simulink model "aerosonde_trim"  (Simulink 7.5)
settings: Solver=ode3  StartTime=0.0  StopTime=60  FixedStep=20e-3  RelTol=1e-6
values from neighbouring files (symbols this model uses):
  aerosonde = aerosonde_data    [aerosonde_initialize.m]    (also in aerosonde_trimlin.m)
  euler_ini = [0;  0.0564; 0]    [aerosonde_trimlin.m]
  fuel_ini = 2    [aerosonde_trimlin.m]
  Omega_ini = 5236*pi/30    (= 548.312637807)    [aerosonde_trimlin.m]
  position_ini = [0; 0; -1000]    [aerosonde_trimlin.m]
  rates_ini = [0; 0; 0]    [aerosonde_trimlin.m]
  velocity_ini = [24.95;   0;   1.4]    [aerosonde_trimlin.m]
libraries: aerolibasang x3, aerolibbdyn x3, aerolibadyn x1, aerolibtransform2 x1, aerolib6dof2 x1, aerolibutil x1, aerolibatmos2 x1
settings Model: Creator=eh3081  LastModifiedBy=eh3081
settings DataIOCC: LimitDataPoints=off  SaveOutput=off  SignalLogging=off  SaveTime=off
settings OptimizationCC: InitFltsAndDblsToZero=on
settings DebuggingCC: SaveWithParameterizedLinksMsg=none  MultiTaskDSMMsg=warning  MultiTaskCondExecSysMsg=none  StrictBusMsg=Warning
settings RTWCC: IncludeERTFirstTime=on
settings GRTTargetCC: TargetFcnLib=ansi_tfl_tmw.mat

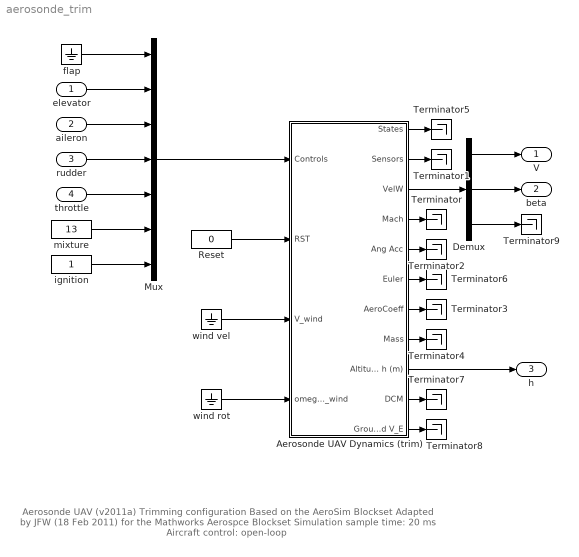
== system aerosonde_trim ==
  note: Aerosonde UAV (v2011a)
      | Trimming configuration
      | Based on the AeroSim Blockset
      | Adapted by JFW (18 Feb 2011) for the Mathworks Aerospce Blockset
      | Simulation sample time: 20 ms
      | Aircraft control: open-loop
  elevator : Inport
  aileron : Inport  Port=2
  rudder : Inport  Port=3
  throttle : Inport  Port=4
  Aerosonde UAV Dynamics (trim) : Subsystem  mask(6-DOF Aerosonde Model){as=aerosonde, Velocities0=velocity_ini, Rates0=rates_ini, Euler0=euler_ini, Position0=position_ini, Fuel0=fuel_ini, Omega0=Omega_ini, GndAlt=0}
      mask prompts: as "Aircraft configuration data:"; Velocities0 "Initial velocity in body axes [u,v,w]: (m/s)"; Rates0 "Initial body rotation rates [p,q,r]: (rad/s)"; Euler0 "Initial Euler orientation [roll, pitch, yaw]: (rad)"; Position0 "Initial position in inertial axes [Xe,Ye,Ze]: (m)"; Fuel0 "Initial fuel mass: (Kg)"; Omega0 "Initial engine speed: (rad/s)"; GndAlt "Ground altitude: (m)"
      mask help:
      | Nonlinear 6-DOF Aerosonde  model with equations of motion in
      | body frame (trim).
      |
      | Version 2011a (18 February 2011)
      |
      | NOTE: the algebraic loop has been removed and the rate set to zero
      |       the wind rate has been set to zero
      mask Help:
      | The block implements the 6-DOF nonlinear Aerosonde model. It is an adaptation of the model provided in the AeroSim blockset. Velocities are computed in body frame.
      | <P><B>Inputs:</B>
      | <LI>Controls = the 4x1 vector of aircraft controls [elevator aileron rudder throttle]. Aerodynamic controls are in radians, throttle is from 0 to 1.</LI>
      | <LI>RST = the integrator reset flag (0 or 1, all integrators on rising edge)
      | <LI>V_wind = the 3x1 vector of background wind speed components in navigation frame [North East Down]</LI>
      | <LI>omega_wind = the 3x1 vector of background wind angular rates in navigation frame [North East Down]</LI>
      | </P>
      | <P><B>Outputs:</B>
      | <LI>States = the 14x1 aircraft state vector [Velocities, Angular rates, Euler angles, Position, Fuel mass, Engine speed].</LI>
      | <LI>Sensors = the 15x1 vector of sensor outputs [GPS Position, GPS Groundspeed, Accelerometers, Gyros, Air data].</LI>
      | <LI>VelW = the 3x1 vector of aircraft velocity in wind axes [Airspeed, sideslip, angle of attack]</LI>
      | <LI>Mach = the Mach number</LI>
      | <LI>Ang Acc = the 3x1 vector of angular accelerations
      | <LI>Euler = the 3x1 vector of Euler angles (roll, pitch, yaw)</LI>
      | <LI>AeroCoeff = the 6x1 vector of aerodynamic coefficients [CD CY CL Cl Cm Cn]</LI>
      | <LI>Mass = the current aircraft mass</LI>
      | <LI>h = the aircraft altitude</LI>
      | </P>
      | <P><B>Parameters:</B>
      | <LI>Aircraft configuration data = structured varaible with aircraft data<BR>
      | obtain by  ``aerosonde=aerosonde_initialize'' for example</LI>
      | <LI>Initial velocities = the 3x1 vector of initial aircraft velocities in body axes [u v w]</LI>
      | <LI>Initial angular rates = the 3x1 vector of initial angular rates [p q r]</LI>
      | <LI>Initial attitude = the 3x1 vector of initial Euler angles [phi theta psi]</LI>
      | <LI>Initial position = the 3x1 vector of initial aircraft location [Lat Lon Alt]</LI>
      | <LI>Initial fuel mass = the initial quantity of fuel on-board the aircraft</LI>
      | <LI>Initial engine speed = the initial engine rotation speed</LI>
      | <LI>Ground altitude = the ground altitude at aircraft location</LI>
      | </P>
      | <P>
      | <I>Version 2010b (26 May 2010)</I>
      | </P>
  Demux : Demux  Outputs=3
  Mux : Mux  Inputs=7
  Reset : Constant  Value=0
  Terminator{,1..9} (10 alike) : Terminator
  flap : Ground
  ignition : Constant
  mixture : Constant  Value=13
  wind rot : Ground
  wind vel : Ground
  V : Outport
  beta : Outport  Port=2
  h : Outport  Port=3
  wires:
  Reset/1 -> Aerosonde UAV Dynamics (trim)/2(RST)
  Demux/3 -> Terminator9/1
  Aerosonde UAV Dynamics (trim)/3(VelW) -> Demux/1
  Aerosonde UAV Dynamics (trim)/4(Mach) -> Terminator/1
  Aerosonde UAV Dynamics (trim)/2(Sensors) -> Terminator1/1
  Aerosonde UAV Dynamics (trim)/5(Ang Acc) -> Terminator2/1
  Aerosonde UAV Dynamics (trim)/7(AeroCoeff) -> Terminator3/1
  Aerosonde UAV Dynamics (trim)/8(Mass) -> Terminator4/1
  Aerosonde UAV Dynamics (trim)/1(States) -> Terminator5/1
  Aerosonde UAV Dynamics (trim)/9("Altitude h (m) ") -> h/1
  wind vel/1 -> Aerosonde UAV Dynamics (trim)/3(V_wind)
  wind rot/1 -> Aerosonde UAV Dynamics (trim)/4(omega_wind)
  Aerosonde UAV Dynamics (trim)/6(Euler) -> Terminator6/1
  Aerosonde UAV Dynamics (trim)/10(DCM) -> Terminator7/1
  Aerosonde UAV Dynamics (trim)/11(Groundspeed V_E) -> Terminator8/1
  Mux/1 -> Aerosonde UAV Dynamics (trim)/1(Controls)
  flap/1 -> Mux/1
  elevator/1 -> Mux/2
  aileron/1 -> Mux/3
  rudder/1 -> Mux/4
  throttle/1 -> Mux/5
  mixture/1 -> Mux/6
  ignition/1 -> Mux/7
  Demux/1 -> V/1
  Demux/2 -> beta/1

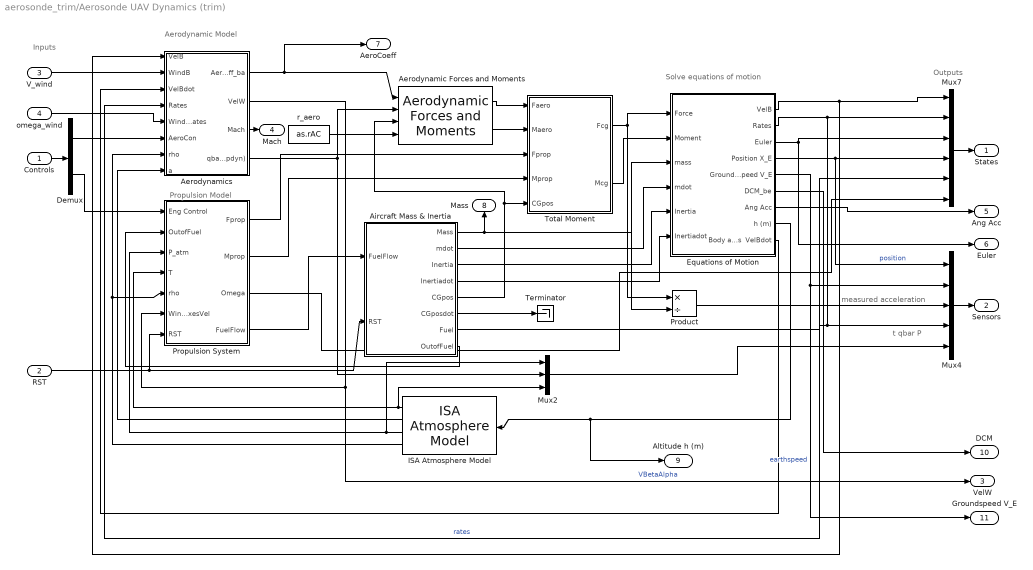
== system aerosonde_trim/Aerosonde UAV Dynamics (trim) ==
  note: Solve equations of motion
  note: Inputs
  note: Outputs
  note: Aerodynamic Model
  note: Propulsion Model
  note: measured acceleration
  note: t qbar P
  Controls : Inport
  RST : Inport  Port=2
  V_wind : Inport  Port=3
  omega_wind : Inport  Port=4
  Aerodynamic Forces and Moments : aerolibadyn/Aerodynamic Forces and Moments   SystemSampleTime=-1  inputAxes=Body  outputForceAxes=Body  outputMomentAxes=Body  S=as.S  b=as.b  cbar=as.c
  Aerodynamics : Subsystem
  Aircraft Mass & Inertia : Subsystem
  Demux : Demux  Outputs=[4,3]
  Equations of Motion : Subsystem
  ISA Atmosphere Model : aerolibatmos2/ISA Atmosphere Model  SystemSampleTime=-1  custom=off  g=9.80665  gamma=1.4  R=287.0531  L=0.0065  h_trop=11000  h_strat=20000  rho0=1.225  P0=101325  T0=288.15
  Mux2 : Mux  Inputs=3
  Mux4 : Mux  Inputs=5
  Mux7 : Mux  Inputs=6
  Product : Product  Inputs=*/  RndMeth=Zero
  Propulsion System : Subsystem  mask(General-aviation propulsion system){OmegaIni=Omega0, RPM=as.RPM, MAP=as.MAP, FuelFlow=as.FuelFlow, Power=as.Power, Jeng=as.Jeng, J=as.J, CT=as.CT, CP=as.CP, Rprop=as.Rprop, Jprop=as.Jprop, TSL=as.TSL}
      mask prompts: OmegaIni "Initial engine speed:"; RPM "Engine RPM vector:"; MAP "Engine MAP vector:"; FuelFlow "Engine fuel flow look-up table:"; Power "Engine power look-up table:"; Jeng "Engine moment of inertia:"; J "Propeller advance ratio vector:"; CT "Propeller coefficient of thrust vector:"; CP "Propeller coefficient of power vector:"; Rprop "Propeller radius:"; Jprop "Propeller moment of inertia:"; TSL "Sea-level temperature:"
      mask help: The block models a general aviation propulsion system including a piston engine and a fixed-pitch propeller.
      mask Help:
      | The block provides a general aviation propulsion system using the AeroSim piston engine and fixed-pitch propeller models.
      | <P><B>Inputs:</B>
      | <LI>Control = the 3x1 engine control vector [Throttle Mixture Ignition]</LI>
      | <LI>OutofFuel = the out-of-fuel flag (0 or 1)</LI>
      | <LI>p = the static pressure at current altitude, in Pa</LI>
      | <LI>T = the air temperature at current altitude, in K</LI>
      | <LI>rho = the air density at current altitude, in kg/m^3</LI>
      | <LI>WindAxesVel = the 3x1 vector of body velocities in wind axes [Airspeed Sideslip Angle-of-attack] in [m/s rad rad]</LI>
      | <LI>RST = the integrator reset flag (rising edge)</LI>
      | </P>
      | <P><B>Output:</B>
      | <LI>Fprop = the 3x1 vector of propulsion system forces applied to the airframe, at the propeller hub location</LI>
      | <LI>Mprop = the 3x1 vector of propulsion system moments applied to the airframe</LI>
      | <LI>Omega = the engine shaft rotation speed, in rad/s</LI>
      | <LI>FuelFlow = the mass fuel flow, in kg/s</LI>
      | <LI>EngCoeff = the 5x1 engine coefficient vector [MAP Airflow Fuelflow BSFC Power] in [kPa kg/s kg/s g/(W*hr) W]</LI>
      | <LI>PropCoeff = the 3x1 propeller coefficient vector [J CT CP]</LI>
      | </P>
      | <P><B>Parameters:</B>
      | <LI>Initial engine speed = the initial value for the engine speed, in rad/s</LI>
      | <LI>RPM vector = the engine speed interpolation vector, in rpm</LI>
      | <LI>MAP vector = the manifold air pressure interpolation vector, in kPa</LI>
      | <LI>Fuel flow = the 2-D look-up table for fuel flow, as function of MAP and RPM, in g/hr</LI>
      | <LI>Power = the 2-D look-up table for power, as function of MAP and RPM, in W</LI>
      | <LI>Engine moment of inertia = the moment of inertia of the rotating engine parts (shaft)</LI>
      | <LI>Advance ratio = the advance ratio vector for interpolation</LI>
      | <LI>Coefficient of thrust = the coefficient of thrust vector for interpolation</LI>
      | <LI>Coefficient of power = the coefficient of power vector for interpolation</LI>
      | <LI>Radius = the propeller radius</LI>
      | <LI>Propeller moment of inertia = the moment of inertia of the propeller</LI>
      | <LI>Sea-level temperature = the ambient temperature for which the above engine look-up tables are given</LI>
      | </P>
  Terminator : Terminator
  Total Moment : Subsystem
  r_aero : Constant  Value=as.rAC
  States : Outport
  Sensors : Outport  Port=2
  VelW : Outport  Port=3
  Mach : Outport  Port=4
  Ang Acc : Outport  Port=5
  Euler : Outport  Port=6
  AeroCoeff : Outport  Port=7
  Mass : Outport  Port=8
  "Altitude h (m) " : Outport  Port=9
  DCM : Outport  Port=10
  Groundspeed V_E : Outport  Port=11
  wires:
  Equations of Motion/3(Euler) -> Euler/1, Mux7/3
  Equations of Motion/7(Ang Acc) -> Ang Acc/1
  RST/1 -> Propulsion System/7(RST), Aircraft Mass & Inertia/2(RST)
  Aircraft Mass & Inertia/8(OutofFuel) -> Propulsion System/2(OutofFuel)
  Aerodynamics/2(VelW) -> Propulsion System/6(WindAxesVel), VelW/1  "VBetaAlpha"
  Propulsion System/3(Omega) -> Mux7/6
  Aircraft Mass & Inertia/7(Fuel) -> Mux7/5
  Mux2/1 -> Mux4/5
  Aerodynamics/4(qbar (pdyn)) -> Mux2/2, Aerodynamic Forces and Moments/2
  Equations of Motion/6(DCM_be) -> DCM/1
  Propulsion System/2(Mprop) -> Total Moment/4(Mprop)
  Propulsion System/1(Fprop) -> Total Moment/3(Fprop)
  Aircraft Mass & Inertia/5(CGpos) -> Total Moment/5(CGpos), Aerodynamic Forces and Moments/3
  Total Moment/2(Mcg) -> Equations of Motion/2(Moment)
  Aircraft Mass & Inertia/1(Mass) -> Mass/1, Equations of Motion/3(mass), Product/2
  Equations of Motion/5(Groundspeed V_E) -> Mux4/2, Groundspeed V_E/1  "earthspeed"
  Controls/1 -> Demux/1
  Mux4/1 -> Sensors/1
  Mux7/1 -> States/1
  Demux/2 -> Propulsion System/1(Eng Control)
  Equations of Motion/1(VelB) -> Mux7/1, Aerodynamics/1(VelB)
  Equations of Motion/2(Rates) -> Aerodynamics/4(Rates), Mux4/4, Mux7/2  "rates"
  Equations of Motion/4(Position X_E) -> Mux7/4, Mux4/1  "position"
  Demux/1 -> Aerodynamics/6(AeroCon)
  Aerodynamics/3(Mach) -> Mach/1
  Aerodynamics/1(AeroCoeff_ba) -> AeroCoeff/1, Aerodynamic Forces and Moments/1
  ISA Atmosphere Model/1 -> Propulsion System/4(T), Mux2/3
  ISA Atmosphere Model/2 -> Aerodynamics/8("a ")
  ISA Atmosphere Model/3 -> Propulsion System/3(P_atm), Mux2/1
  ISA Atmosphere Model/4 -> Aerodynamics/7(rho), Propulsion System/5(rho)
  Equations of Motion/8(h (m)) -> ISA Atmosphere Model/1, "Altitude h (m) "/1
  Aircraft Mass & Inertia/2(mdot) -> Equations of Motion/4(mdot)
  r_aero/1 -> Aerodynamic Forces and Moments/4
  Aerodynamic Forces and Moments/1 -> Total Moment/1(Faero)
  Aerodynamic Forces and Moments/2 -> Total Moment/2(Maero)
  Total Moment/1(Fcg) -> Equations of Motion/1(Force), Product/1
  Aircraft Mass & Inertia/3(Inertia) -> Equations of Motion/5(Inertia)
  Aircraft Mass & Inertia/4(Inertiadot) -> Equations of Motion/6(Inertiadot)
  Aircraft Mass & Inertia/6(CGposdot) -> Terminator/1
  Product/1 -> Mux4/3
  Propulsion System/4(FuelFlow) -> Aircraft Mass & Inertia/1(FuelFlow)
  Equations of Motion/9(Body accns  VelBdot) -> Aerodynamics/3(VelBdot)
  omega_wind/1 -> Aerodynamics/5(WindRates)
  V_wind/1 -> Aerodynamics/2(WindB)

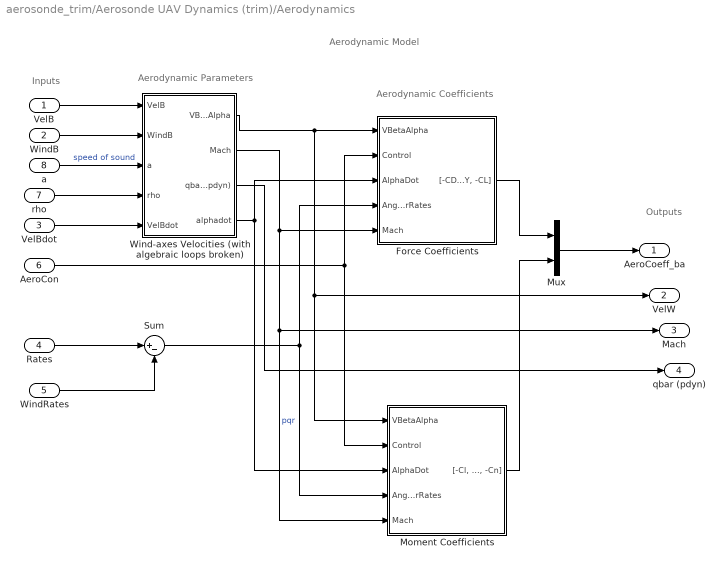
== system aerosonde_trim/Aerosonde UAV Dynamics (trim)/Aerodynamics ==
  note: Inputs
  note: Outputs
  note: Aerodynamic Parameters
  note: Aerodynamic Coefficients
  note: Aerodynamic Model
  VelB : Inport  PortDimensions=[3 1]
  WindB : Inport  Port=2  PortDimensions=[3 1]
  VelBdot : Inport  Port=3
  Rates : Inport  Port=4  PortDimensions=[3 1]
  WindRates : Inport  Port=5  PortDimensions=[3 1]
  AeroCon : Inport  Port=6  PortDimensions=[4 1]
  rho : Inport  Port=7  PortDimensions=1
  "a " : Inport  Port=8  PortDimensions=1
  Force Coefficients : Subsystem
  Moment Coefficients : Subsystem
  Mux : Mux  Inputs=2
  Sum : Sum  Inputs=|+-  SaturateOnIntegerOverflow=on  InputSameDT=on  OutDataTypeStr=Inherit: Same as first input
  Wind-axes Velocities (with algebraic loops broken) : Subsystem
  AeroCoeff_ba : Outport
  VelW : Outport  Port=2
  Mach : Outport  Port=3
  qbar (pdyn) : Outport  Port=4
  wires:
  Sum/1 -> Force Coefficients/4(AngularRates), Moment Coefficients/4(AngularRates)  "pqr"
  WindRates/1 -> Sum/2
  Rates/1 -> Sum/1
  Wind-axes Velocities (with algebraic loops broken)/3(qbar (pdyn)) -> qbar (pdyn)/1
  Wind-axes Velocities (with algebraic loops broken)/2(Mach) -> Mach/1, Force Coefficients/5(Mach), Moment Coefficients/5(Mach)
  AeroCon/1 -> Force Coefficients/2(Control), Moment Coefficients/2(Control)
  Wind-axes Velocities (with algebraic loops broken)/1(VBetaAlpha) -> Force Coefficients/1(VBetaAlpha), VelW/1, Moment Coefficients/1(VBetaAlpha)
  "a "/1 -> Wind-axes Velocities (with algebraic loops broken)/3(a)  "speed of sound"
  VelB/1 -> Wind-axes Velocities (with algebraic loops broken)/1(VelB)
  rho/1 -> Wind-axes Velocities (with algebraic loops broken)/4(rho)
  Force Coefficients/1("[-CD, CY, -CL]") -> Mux/1
  Moment Coefficients/1("[-Cl, Cm, -Cn]") -> Mux/2
  Mux/1 -> AeroCoeff_ba/1
  WindB/1 -> Wind-axes Velocities (with algebraic loops broken)/2(WindB)
  Wind-axes Velocities (with algebraic loops broken)/4(alphadot) -> Moment Coefficients/3(AlphaDot), Force Coefficients/3(AlphaDot)
  VelBdot/1 -> Wind-axes Velocities (with algebraic loops broken)/5(VelBdot)

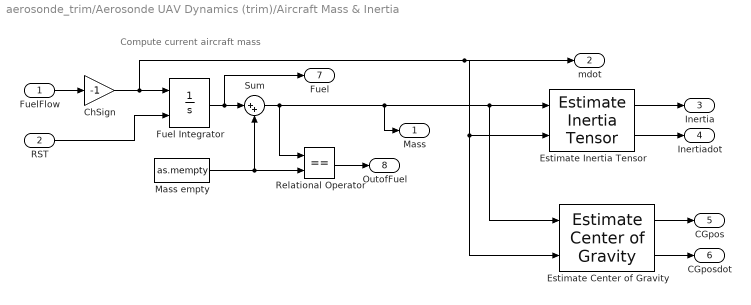
== system aerosonde_trim/Aerosonde UAV Dynamics (trim)/Aircraft Mass & Inertia ==
  note: Compute current aircraft mass
  FuelFlow : Inport  PortDimensions=1
  RST : Inport  Port=2  PortDimensions=1
  ChSign : Gain  Gain=-1  SaturateOnIntegerOverflow=on  OutDataTypeStr=Inherit: Same as input  ParamDataTypeStr=Inherit: Same as input
  Estimate Center of Gravity : aerolibbdyn/Estimate Center of Gravity  SystemSampleTime=-1  fmass=as.mgross  emass=as.mempty  fcg=as.CGgross  ecg=as.CGempty
  Estimate Inertia Tensor : aerolibbdyn/Estimate Inertia Tensor  SystemSampleTime=-1  fmass=as.mgross  emass=as.mempty  fI=as.J_gross  eI=as.J_empty
  Fuel Integrator : Integrator  ExternalReset=rising  InitialCondition=Fuel0  LimitOutput=on  UpperSaturationLimit=as.mgross-as.mempty  LowerSaturationLimit=0
  Mass empty : Constant  Value=as.mempty
  Relational Operator : RelationalOperator  Operator===  InputSameDT=on
  Sum : Sum  Inputs=|++  SaturateOnIntegerOverflow=on  InputSameDT=on  OutDataTypeStr=Inherit: Same as first input
  Mass : Outport
  mdot : Outport  Port=2
  Inertia : Outport  Port=3
  Inertiadot : Outport  Port=4
  CGpos : Outport  Port=5
  CGposdot : Outport  Port=6
  Fuel : Outport  Port=7
  OutofFuel : Outport  Port=8
  wires:
  Relational Operator/1 -> OutofFuel/1
  FuelFlow/1 -> ChSign/1
  ChSign/1 -> Fuel Integrator/1, mdot/1, Estimate Inertia Tensor/2, Estimate Center of Gravity/2
  RST/1 -> Fuel Integrator/2
  Fuel Integrator/1 -> Fuel/1, Sum/1
  Mass empty/1 -> Relational Operator/2, Sum/2
  Sum/1 -> Mass/1, Estimate Inertia Tensor/1, Estimate Center of Gravity/1, Relational Operator/1
  Estimate Inertia Tensor/1 -> Inertia/1
  Estimate Inertia Tensor/2 -> Inertiadot/1
  Estimate Center of Gravity/1 -> CGpos/1
  Estimate Center of Gravity/2 -> CGposdot/1

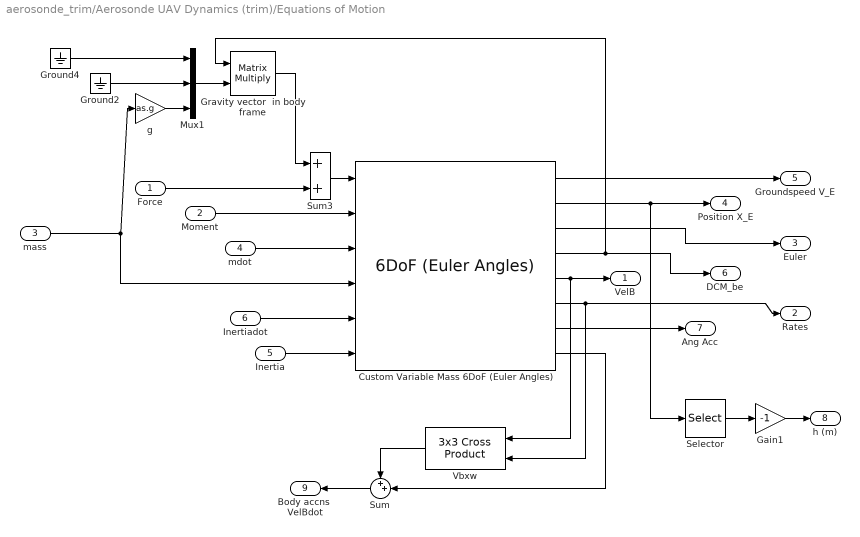
== system aerosonde_trim/Aerosonde UAV Dynamics (trim)/Equations of Motion ==
  Force : Inport  PortDimensions=3
  Moment : Inport  Port=2  PortDimensions=3
  mass : Inport  Port=3  PortDimensions=1
  mdot : Inport  Port=4  PortDimensions=1
  Inertia : Inport  Port=5  PortDimensions=[3,3]
  Inertiadot : Inport  Port=6  PortDimensions=[3,3]
  Custom Variable Mass 6DoF (Euler Angles) : aerolib6dof2/6DoF (Euler Angles)  SystemSampleTime=-1  units=Metric (MKS)  mtype=Custom Variable  rep=Euler Angles  xme_0=Position0  Vm_0=Velocities0  eul_0=Euler0  pm_0=Rates0  mass_0=1.0  mass_e=0  mass_f=0  inertia=eye(3)  inertia_e=eye(3)  inertia_f=eye(3)  k_quat=1.0
  Gain1 : Gain  Gain=-1
  "Gravity vector  in body frame " : Product  Multiplication=Matrix(*)  SaturateOnIntegerOverflow=on  InputSameDT=on  OutDataTypeStr=Inherit: Same as first input
  Ground2 : Ground
  Ground4 : Ground
  Mux1 : Mux  Inputs=3
  Selector : Selector  InputPortWidth=3  IndexOptions=Index vector (dialog)  Indices=3  OutputSizes=1
  Sum : Sum  Inputs=++|  SaturateOnIntegerOverflow=on
  Sum3 : Sum  SaturateOnIntegerOverflow=on  InputSameDT=on  OutDataTypeStr=Inherit: Same as first input
  Vbxw : aerolibutil/3x3 Cross Product  SystemSampleTime=-1
  g : Gain  Gain=as.g
  VelB : Outport
  Rates : Outport  Port=2
  Euler : Outport  Port=3
  Position X_E : Outport  Port=4
  Groundspeed V_E : Outport  Port=5
  DCM_be : Outport  Port=6
  Ang Acc : Outport  Port=7
  h (m) : Outport  Port=8
  Body accns  VelBdot : Outport  Port=9
  wires:
  Moment/1 -> Custom Variable Mass 6DoF (Euler Angles)/2
  Force/1 -> Sum3/2
  Mux1/1 -> "Gravity vector  in body frame "/2
  Custom Variable Mass 6DoF (Euler Angles)/4 -> "Gravity vector  in body frame "/1, DCM_be/1
  mass/1 -> g/1, Custom Variable Mass 6DoF (Euler Angles)/4
  Ground2/1 -> Mux1/2
  Ground4/1 -> Mux1/1
  Custom Variable Mass 6DoF (Euler Angles)/5 -> VelB/1, Vbxw/1
  Custom Variable Mass 6DoF (Euler Angles)/1 -> Groundspeed V_E/1
  Custom Variable Mass 6DoF (Euler Angles)/2 -> Position X_E/1, Selector/1
  Custom Variable Mass 6DoF (Euler Angles)/3 -> Euler/1
  "Gravity vector  in body frame "/1 -> Sum3/1
  g/1 -> Mux1/3
  Sum3/1 -> Custom Variable Mass 6DoF (Euler Angles)/1
  Selector/1 -> Gain1/1
  Gain1/1 -> h (m)/1
  Inertiadot/1 -> Custom Variable Mass 6DoF (Euler Angles)/5
  mdot/1 -> Custom Variable Mass 6DoF (Euler Angles)/3
  Inertia/1 -> Custom Variable Mass 6DoF (Euler Angles)/6
  Custom Variable Mass 6DoF (Euler Angles)/6 -> Rates/1, Vbxw/2
  Custom Variable Mass 6DoF (Euler Angles)/7 -> Ang Acc/1
  Custom Variable Mass 6DoF (Euler Angles)/8 -> Sum/2
  Sum/1 -> Body accns  VelBdot/1
  Vbxw/1 -> Sum/1

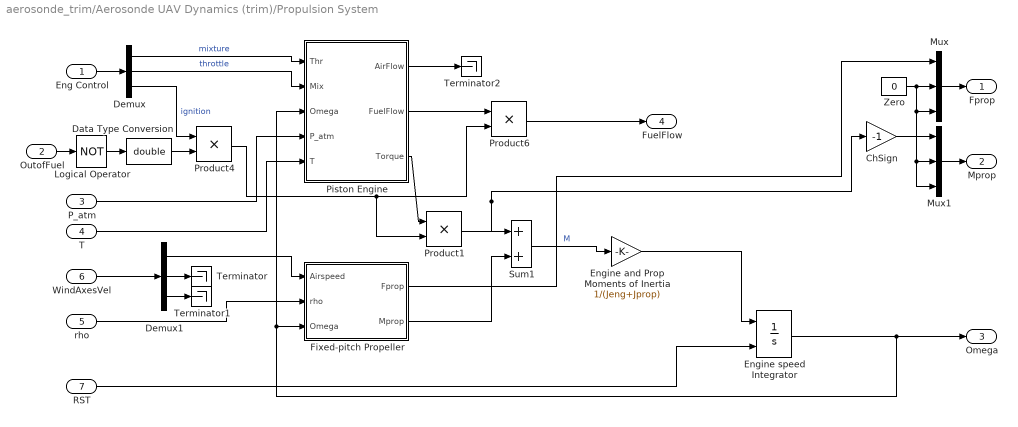
== system aerosonde_trim/Aerosonde UAV Dynamics (trim)/Propulsion System ==
  Eng Control : Inport  PortDimensions=[3 1]
  OutofFuel : Inport  Port=2  PortDimensions=1
  P_atm : Inport  Port=3  OutDataTypeStr=double  PortDimensions=1  DataType=double
  T : Inport  Port=4  OutDataTypeStr=double  PortDimensions=1  DataType=double
  rho : Inport  Port=5  OutDataTypeStr=double  PortDimensions=1  DataType=double
  WindAxesVel : Inport  Port=6  PortDimensions=[3 1]
  RST : Inport  Port=7  OutDataTypeStr=double  PortDimensions=1  DataType=double
  ChSign : Gain  Gain=-1  SaturateOnIntegerOverflow=on  OutDataTypeStr=Inherit: Same as input  ParamDataTypeStr=Inherit: Same as input
  Data Type Conversion : DataTypeConversion  OutDataTypeStr=double  OutDataTypeMode=double  SaturateOnIntegerOverflow=on  RndMeth=Zero
  Demux : Demux  Outputs=3
  Demux1 : Demux  Outputs=3
  Engine and Prop Moments of Inertia : Gain  Gain=1/(Jeng+Jprop)  SaturateOnIntegerOverflow=on  OutDataTypeStr=Inherit: Same as input  ParamDataTypeStr=Inherit: Same as input
  Engine speed Integrator : Integrator  ExternalReset=rising  InitialCondition=OmegaIni  LimitOutput=on  LowerSaturationLimit=0
  Fixed-pitch Propeller : Subsystem
  Logical Operator : Logic  Operator=NOT
  Mux : Mux  Inputs=3
  Mux1 : Mux  Inputs=3
  Piston Engine : Subsystem  mask(Piston Engine){RPM=RPM, MAP=MAP, fflow=FuelFlow, Power=Power, TSL=TSL}
      mask prompts: RPM "RPM vector:"; MAP "MAP vector:"; fflow "Fuel flow 2-D look-up table:"; Power "Power 2-D look-up table:"; TSL "Sea-level temperature:"
      mask help: The piston engine model computes the engine parameters at current throttle setting, engine rpm, and altitude.
      mask Help:
      | The block provides a piston engine model based on look-up tables for manifold pressure, engine speed (rpm), fuel flow and power.
      | <P><B>Inputs:</B>
      | <LI>Thr = the throttle command (as a fraction of atmospheric pressure)</LI>
      | <LI>Mix = the air to fuel mixture ratio</LI>
      | <LI>Omega = the engine shaft rotation speed</LI>
      | <LI>p = the atmospheric pressure, in Pa</LI>
      | <LI>T = the atmospheric temperature, in K</LI>
      | </P>
      | <P><B>Output:</B>
      | <LI>MAP = the manifold air pressure, in kPa</LI>
      | <LI>AirFlow = the mass air flow, in kg/s</LI>
      | <LI>FuelFlow = the mass fuel flow, in kg/s</LI>
      | <LI>BSFC = the brake-specific fuel consumption, in g/(W*hr)</LI>
      | <LI>Power = the engine power, in W</LI>
      | <LI>Torque = the engine shaft torque, in N*m</LI>
      | </P>
      | <P><B>Parameters:</B>
      | <LI>RPM vector = the engine speed interpolation vector, in rpm</LI>
      | <LI>MAP vector = the manifold air pressure interpolation vector, in kPa</LI>
      | <LI>Fuel flow = the 2-D look-up table for fuel flow, as function of MAP and RPM, in g/hr</LI>
      | <LI>Power = the 2-D look-up table for power, as function of MAP and RPM, in W</LI>
      | <LI>Sea-level temperature = the ambient temperature for which the above engine look-up tables are given</LI>
      | </P>
  Product1 : Product  SaturateOnIntegerOverflow=on  InputSameDT=on  OutDataTypeStr=Inherit: Same as first input
  Product4 : Product  SaturateOnIntegerOverflow=on  InputSameDT=on  OutDataTypeStr=Inherit: Same as first input
  Product6 : Product  SaturateOnIntegerOverflow=on  InputSameDT=on  OutDataTypeStr=Inherit: Same as first input
  Sum1 : Sum  SaturateOnIntegerOverflow=on  InputSameDT=on  OutDataTypeStr=Inherit: Same as first input
  Terminator : Terminator
  Terminator1 : Terminator
  Terminator2 : Terminator
  Zero : Constant  Value=0
  Fprop : Outport
  Mprop : Outport  Port=2
  Omega : Outport  Port=3
  FuelFlow : Outport  Port=4
  wires:
  Data Type Conversion/1 -> Product4/2
  Eng Control/1 -> Demux/1
  WindAxesVel/1 -> Demux1/1
  Demux1/2 -> Terminator/1
  Demux1/3 -> Terminator1/1
  Demux1/1 -> Fixed-pitch Propeller/1(Airspeed)
  rho/1 -> Fixed-pitch Propeller/2(rho)
  OutofFuel/1 -> Logical Operator/1
  Product4/1 -> Product6/2, Product1/2
  Product1/1 -> Sum1/1, ChSign/1
  Fixed-pitch Propeller/2(Mprop) -> Sum1/2
  Sum1/1 -> Engine and Prop Moments of Inertia/1  "M"
  RST/1 -> Engine speed Integrator/2
  Engine speed Integrator/1 -> Fixed-pitch Propeller/3(Omega), Piston Engine/3(Omega), Omega/1
  Piston Engine/3(Torque) -> Product1/1
  Zero/1 -> Mux/2, Mux/3, Mux1/3, Mux1/2
  Fixed-pitch Propeller/1(Fprop) -> Mux/1
  ChSign/1 -> Mux1/1
  Mux/1 -> Fprop/1
  Mux1/1 -> Mprop/1
  Logical Operator/1 -> Data Type Conversion/1
  Demux/3 -> Product4/1  "ignition"
  Demux/1 -> Piston Engine/1(Thr)  "mixture"
  Demux/2 -> Piston Engine/2(Mix)  "throttle"
  P_atm/1 -> Piston Engine/4(P_atm)
  T/1 -> Piston Engine/5(T)
  Engine and Prop Moments of Inertia/1 -> Engine speed Integrator/1
  Piston Engine/2(FuelFlow) -> Product6/1
  Product6/1 -> FuelFlow/1
  Piston Engine/1(AirFlow) -> Terminator2/1

== system aerosonde_trim/Aerosonde UAV Dynamics (trim)/Total Moment ==
  note: Total moments at CG location
  note: Sum forces and moments
  Faero : Inport  PortDimensions=3
  Maero : Inport  Port=2  PortDimensions=3
  Fprop : Inport  Port=3  PortDimensions=3
  Mprop : Inport  Port=4  PortDimensions=3
  CGpos : Inport  Port=5  PortDimensions=3
  Moments about CG  due to Propulsion   Forces : aerolibbdyn/Moments about CG  due to Forces  SystemSampleTime=-1
  Sum1 : Sum  Inputs=+++  SaturateOnIntegerOverflow=on  InputSameDT=on  OutDataTypeStr=Inherit: Same as first input
  Total forces  (excluding g) : Sum  SaturateOnIntegerOverflow=on  InputSameDT=on  OutDataTypeStr=Inherit: Same as first input
  r_prop : Constant  Value=as.rHub  OutDataTypeStr=double  OutDataTypeMode=double
  Fcg : Outport
  Mcg : Outport  Port=2
  wires:
  CGpos/1 -> Moments about CG  due to Propulsion   Forces/2
  r_prop/1 -> Moments about CG  due to Propulsion   Forces/3
  Sum1/1 -> Mcg/1
  Mprop/1 -> Sum1/3
  Fprop/1 -> Moments about CG  due to Propulsion   Forces/1, Total forces  (excluding g)/2
  Faero/1 -> Total forces  (excluding g)/1
  Total forces  (excluding g)/1 -> Fcg/1
  Moments about CG  due to Propulsion   Forces/1 -> Sum1/1
  Maero/1 -> Sum1/2

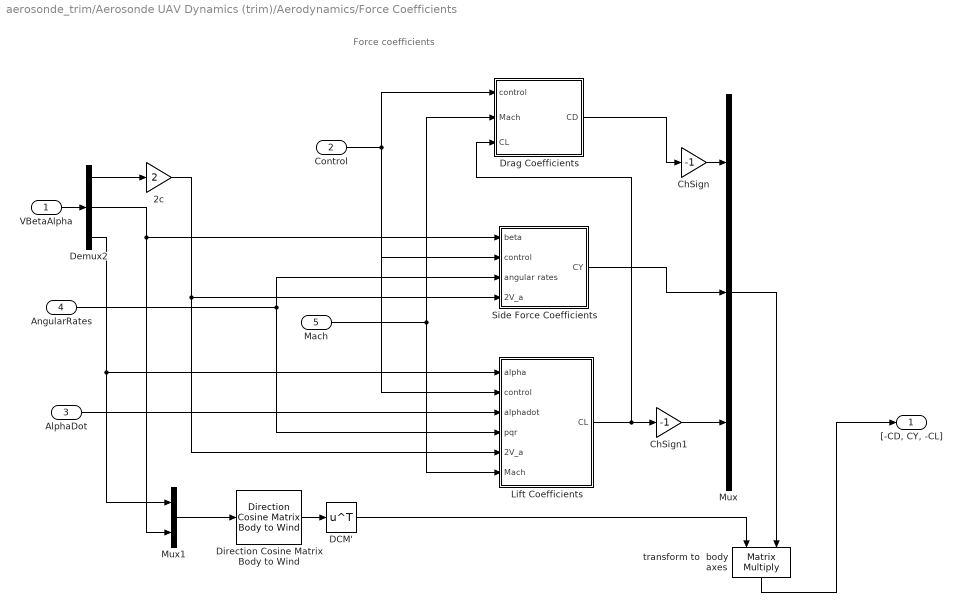
== system aerosonde_trim/Aerosonde UAV Dynamics (trim)/Aerodynamics/Force Coefficients ==
  note: Force coefficients
  VBetaAlpha : Inport  PortDimensions=[3 1]
  Control : Inport  Port=2  PortDimensions=[4 1]
  AlphaDot : Inport  Port=3
  AngularRates : Inport  Port=4  PortDimensions=[3 1]
  Mach : Inport  Port=5  PortDimensions=1
  2c : Gain  Gain=2  SaturateOnIntegerOverflow=on  OutDataTypeStr=Inherit: Same as input  ParamDataTypeStr=Inherit: Same as input
  ChSign : Gain  Gain=-1  SaturateOnIntegerOverflow=on  OutDataTypeStr=Inherit: Same as input  ParamDataTypeStr=Inherit: Same as input
  ChSign1 : Gain  Gain=-1  SaturateOnIntegerOverflow=on  OutDataTypeStr=Inherit: Same as input  ParamDataTypeStr=Inherit: Same as input
  DCM' : Math  Operator=transpose  SaturateOnIntegerOverflow=on
  Demux2 : Demux  Outputs=3
  Direction Cosine Matrix Body to Wind : aerolibtransform2/Direction Cosine Matrix Body to Wind  SystemSampleTime=-1
  Drag Coefficients : Subsystem
  Lift Coefficients : Subsystem
  Mux : Mux  Inputs=3
  Mux1 : Mux  Inputs=2
  Side Force Coefficients : Subsystem
  transform to  body axes : Product  Inputs=**  Multiplication=Matrix(*)  SaturateOnIntegerOverflow=on  InputSameDT=on  OutDataTypeStr=Inherit: Same as first input
  "[-CD, CY, -CL]" : Outport
  wires:
  2c/1 -> Lift Coefficients/5(2V_a), Side Force Coefficients/4(2V_a)
  Demux2/3 -> Mux1/1, Lift Coefficients/1(alpha)
  Control/1 -> Drag Coefficients/1(control), Side Force Coefficients/2(control), Lift Coefficients/2(control)
  AlphaDot/1 -> Lift Coefficients/3(alphadot)
  AngularRates/1 -> Lift Coefficients/4(pqr), Side Force Coefficients/3(angular rates)
  Mach/1 -> Lift Coefficients/6(Mach), Drag Coefficients/2(Mach)
  Lift Coefficients/1(CL) -> ChSign1/1, Drag Coefficients/3(CL)
  Drag Coefficients/1(CD) -> ChSign/1
  Side Force Coefficients/1(CY) -> Mux/2
  ChSign/1 -> Mux/1
  ChSign1/1 -> Mux/3
  VBetaAlpha/1 -> Demux2/1
  Demux2/1 -> 2c/1
  Demux2/2 -> Side Force Coefficients/1(beta), Mux1/2
  transform to  body axes/1 -> "[-CD, CY, -CL]"/1
  Direction Cosine Matrix Body to Wind/1 -> DCM'/1
  Mux/1 -> transform to  body axes/2
  DCM'/1 -> transform to  body axes/1
  Mux1/1 -> Direction Cosine Matrix Body to Wind/1

== system aerosonde_trim/Aerosonde UAV Dynamics (trim)/Aerodynamics/Moment Coefficients ==
  note: Moment coefficients
  VBetaAlpha : Inport  PortDimensions=[3 1]
  Control : Inport  Port=2  PortDimensions=[4 1]
  AlphaDot : Inport  Port=3
  AngularRates : Inport  Port=4  PortDimensions=[3 1]
  Mach : Inport  Port=5  PortDimensions=1
  2c : Gain  Gain=2  SaturateOnIntegerOverflow=on  OutDataTypeStr=Inherit: Same as input  ParamDataTypeStr=Inherit: Same as input
  Demux1 : Demux  Outputs=3
  Mux : Mux  Inputs=3
  Pitch Moment Coefficients : Subsystem
  Roll Moment Coefficients : Subsystem
  Yaw Moment Coefficients : Subsystem
  "[-Cl, Cm, -Cn]" : Outport
  wires:
  Roll Moment Coefficients/1(Cl) -> Mux/1
  Pitch Moment Coefficients/1(Cm) -> Mux/2
  Mux/1 -> "[-Cl, Cm, -Cn]"/1
  AngularRates/1 -> Pitch Moment Coefficients/4(pqr), Yaw Moment Coefficients/3(angular rates), Roll Moment Coefficients/3(angular rates)
  AlphaDot/1 -> Pitch Moment Coefficients/3(alphadot)
  Control/1 -> Pitch Moment Coefficients/2(control), Yaw Moment Coefficients/2(control), Roll Moment Coefficients/2(control)
  Demux1/1 -> 2c/1
  2c/1 -> Roll Moment Coefficients/4(2V), Yaw Moment Coefficients/4(2V_a), Pitch Moment Coefficients/5(2V_a)
  VBetaAlpha/1 -> Demux1/1
  Yaw Moment Coefficients/1(Cn) -> Mux/3
  Mach/1 -> Pitch Moment Coefficients/6(Mach)
  Demux1/3 -> Pitch Moment Coefficients/1(alpha)
  Demux1/2 -> Roll Moment Coefficients/1(beta), Yaw Moment Coefficients/1(beta)

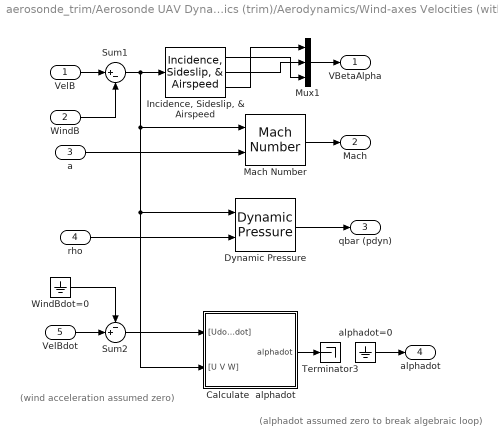
== system aerosonde_trim/Aerosonde UAV Dynamics (trim)/Aerodynamics/Wind-axes Velocities (with algebraic loops broken) ==
  note: (wind acceleration
      |  assumed zero)
  note: (alphadot assumed
      | zero to break
      | algebraic loop)
  VelB : Inport
  WindB : Inport  Port=2
  a : Inport  Port=3
  rho : Inport  Port=4
  VelBdot : Inport  Port=5
  Calculate  alphadot : Subsystem
  Dynamic Pressure : aerolibasang/Dynamic Pressure  SystemSampleTime=-1
  "Incidence, Sideslip, & Airspeed" : aerolibasang/Incidence, Sideslip, & Airspeed  SystemSampleTime=-1
  Mach Number : aerolibasang/Mach Number  SystemSampleTime=-1
  Mux1 : Mux  Inputs=3
  Sum1 : Sum  Inputs=|+-  SaturateOnIntegerOverflow=on  InputSameDT=on  OutDataTypeStr=Inherit: Same as first input
  Sum2 : Sum  Inputs=-+|  SaturateOnIntegerOverflow=on  InputSameDT=on  OutDataTypeStr=Inherit: Same as first input
  Terminator3 : Terminator
  WindBdot=0 : Ground
  alphadot=0 : Ground
  VBetaAlpha : Outport
  Mach : Outport  Port=2
  qbar (pdyn) : Outport  Port=3
  alphadot : Outport  Port=4
  wires:
  Sum1/1 -> "Incidence, Sideslip, & Airspeed"/1, Mach Number/1, Dynamic Pressure/1, Calculate  alphadot/2("[U V W]")
  "Incidence, Sideslip, & Airspeed"/3 -> Mux1/1
  Mux1/1 -> VBetaAlpha/1
  VelB/1 -> Sum1/1
  WindB/1 -> Sum1/2
  Mach Number/1 -> Mach/1
  a/1 -> Mach Number/2
  rho/1 -> Dynamic Pressure/2
  Dynamic Pressure/1 -> qbar (pdyn)/1
  "Incidence, Sideslip, & Airspeed"/1 -> Mux1/3
  "Incidence, Sideslip, & Airspeed"/2 -> Mux1/2
  VelBdot/1 -> Sum2/2
  Sum2/1 -> Calculate  alphadot/1("[Udot Vdot Wdot]")
  WindBdot=0/1 -> Sum2/1
  Calculate  alphadot/1(alphadot) -> Terminator3/1
  alphadot=0/1 -> alphadot/1

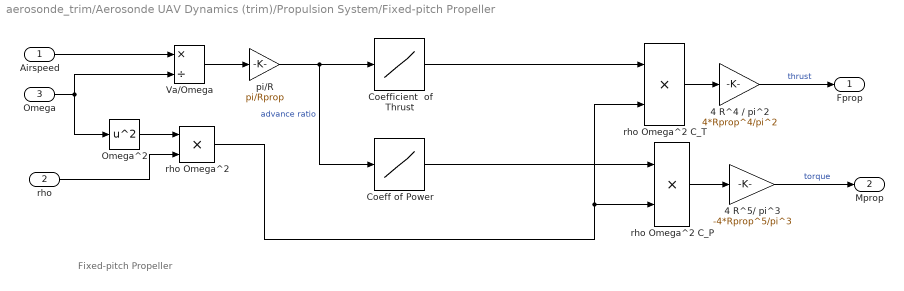
== system aerosonde_trim/Aerosonde UAV Dynamics (trim)/Propulsion System/Fixed-pitch Propeller ==
  note: Fixed-pitch
      | Propeller
  Airspeed : Inport  OutDataTypeStr=double  PortDimensions=1  DataType=double
  rho : Inport  Port=2  OutDataTypeStr=double  PortDimensions=1  DataType=double
  Omega : Inport  Port=3  OutDataTypeStr=double  PortDimensions=1  DataType=double
  4 R^4 / pi^2 : Gain  Gain=4*Rprop^4/pi^2  SaturateOnIntegerOverflow=on  OutDataTypeStr=Inherit: Same as input  ParamDataTypeStr=Inherit: Same as input
  4 R^5/ pi^3 : Gain  Gain=-4*Rprop^5/pi^3  SaturateOnIntegerOverflow=on  OutDataTypeStr=Inherit: Same as input  ParamDataTypeStr=Inherit: Same as input
  Coeff of Power : Lookup  InputValues=J  Table=CP  SaturateOnIntegerOverflow=on
  Coefficient  of Thrust : Lookup  InputValues=J  Table=CT  SaturateOnIntegerOverflow=on
  Omega^2 : Math  Operator=square  SaturateOnIntegerOverflow=on
  Va/Omega : Product  Inputs=*/  SaturateOnIntegerOverflow=on  InputSameDT=on  OutDataTypeStr=Inherit: Same as first input
  pi/R : Gain  Gain=pi/Rprop  SaturateOnIntegerOverflow=on  OutDataTypeStr=Inherit: Same as input  ParamDataTypeStr=Inherit: Same as input
  "rho Omega^2 " : Product  SaturateOnIntegerOverflow=on  InputSameDT=on  OutDataTypeStr=Inherit: Same as first input
  rho Omega^2 C_P : Product  SaturateOnIntegerOverflow=on  InputSameDT=on  OutDataTypeStr=Inherit: Same as first input
  rho Omega^2 C_T : Product  SaturateOnIntegerOverflow=on  InputSameDT=on  OutDataTypeStr=Inherit: Same as first input
  Fprop : Outport
  Mprop : Outport  Port=2
  wires:
  Coeff of Power/1 -> rho Omega^2 C_P/1
  Omega/1 -> Omega^2/1, Va/Omega/2
  Va/Omega/1 -> pi/R/1
  Coefficient  of Thrust/1 -> rho Omega^2 C_T/1
  rho Omega^2 C_T/1 -> 4 R^4 / pi^2/1
  rho Omega^2 C_P/1 -> 4 R^5/ pi^3/1
  pi/R/1 -> Coefficient  of Thrust/1, Coeff of Power/1  "advance ratio"
  Airspeed/1 -> Va/Omega/1
  4 R^4 / pi^2/1 -> Fprop/1  "thrust"
  4 R^5/ pi^3/1 -> Mprop/1  "torque"
  rho/1 -> "rho Omega^2 "/2
  Omega^2/1 -> "rho Omega^2 "/1
  "rho Omega^2 "/1 -> rho Omega^2 C_T/2, rho Omega^2 C_P/2

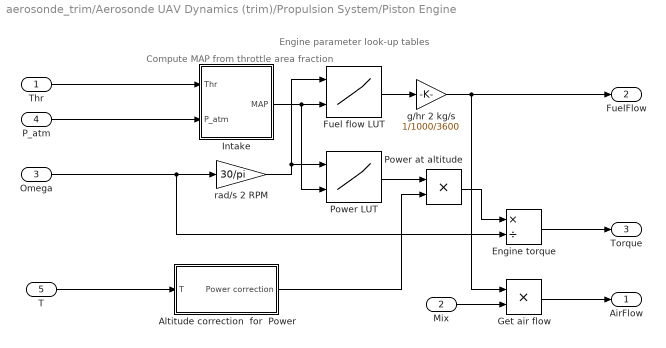
== system aerosonde_trim/Aerosonde UAV Dynamics (trim)/Propulsion System/Piston Engine ==
  note: Engine parameter
      | look-up tables
  note: Compute MAP from
      | throttle area fraction
  Thr : Inport  OutDataTypeStr=double  PortDimensions=1  DataType=double
  Mix : Inport  Port=2  OutDataTypeStr=double  PortDimensions=1  DataType=double
  Omega : Inport  Port=3  OutDataTypeStr=double  PortDimensions=1  DataType=double
  P_atm : Inport  Port=4  OutDataTypeStr=double  PortDimensions=1  DataType=double
  T : Inport  Port=5  OutDataTypeStr=double  PortDimensions=1  DataType=double
  Altitude correction  for  Power : Subsystem
  Engine torque : Product  Inputs=*/  SaturateOnIntegerOverflow=on  InputSameDT=on  OutDataTypeStr=Inherit: Same as first input
  Fuel flow LUT : Lookup2D  RowIndex=RPM  ColumnIndex=MAP  Table=fflow  SaturateOnIntegerOverflow=on  InputSameDT=on
  Get air flow : Product  SaturateOnIntegerOverflow=on  InputSameDT=on  OutDataTypeStr=Inherit: Same as first input
  Intake : Subsystem
  Power LUT : Lookup2D  RowIndex=RPM  ColumnIndex=MAP  Table=Power  SaturateOnIntegerOverflow=on  InputSameDT=on
  Power at altitude : Product  SaturateOnIntegerOverflow=on  InputSameDT=on  OutDataTypeStr=Inherit: Same as first input
  g/hr 2 kg/s : Gain  Gain=1/1000/3600  SaturateOnIntegerOverflow=on  OutDataTypeStr=Inherit: Same as input  ParamDataTypeStr=Inherit: Same as input
  rad/s 2 RPM : Gain  Gain=30/pi  SaturateOnIntegerOverflow=on  OutDataTypeStr=Inherit: Same as input  ParamDataTypeStr=Inherit: Same as input
  AirFlow : Outport
  FuelFlow : Outport  Port=2
  Torque : Outport  Port=3
  wires:
  P_atm/1 -> Intake/2(P_atm)
  Thr/1 -> Intake/1(Thr)
  Engine torque/1 -> Torque/1
  Fuel flow LUT/1 -> g/hr 2 kg/s/1
  Power at altitude/1 -> Engine torque/1
  Altitude correction  for  Power/1(Power correction) -> Power at altitude/2
  Power LUT/1 -> Power at altitude/1
  T/1 -> Altitude correction  for  Power/1(T)
  rad/s 2 RPM/1 -> Power LUT/1, Fuel flow LUT/1
  Omega/1 -> Engine torque/2, rad/s 2 RPM/1
  g/hr 2 kg/s/1 -> FuelFlow/1, Get air flow/1
  Intake/1(MAP) -> Fuel flow LUT/2, Power LUT/2
  Mix/1 -> Get air flow/2
  Get air flow/1 -> AirFlow/1

== system aerosonde_trim/Aerosonde UAV Dynamics (trim)/Aerodynamics/Force Coefficients/Drag Coefficients ==
  note: Drag coefficient
  control : Inport
  Mach : Inport  Port=2
  CL : Inport  Port=3  PortDimensions=1
  (CL-CL0)^2/(pi e AR) : Gain  Gain=1/as.pieaR  Multiplication=Matrix(K*u)  SaturateOnIntegerOverflow=on  OutDataTypeStr=Inherit: Same as input  ParamDataTypeStr=Inherit: Same as input
  Abs4 : Abs  SaturateOnIntegerOverflow=on
  CDM : Gain  Gain=as.CDM  SaturateOnIntegerOverflow=on  OutDataTypeStr=Inherit: Same as input  ParamDataTypeStr=Inherit: Same as input
  CDdf : Gain  Gain=[as.CDdf, as.CDde, as.CDda, as.CDdr]  Multiplication=Matrix(K*u)  SaturateOnIntegerOverflow=on  OutDataTypeStr=Inherit: Same as input  ParamDataTypeStr=Inherit: Same as input
  CL min drag : Constant  Value=as.CLmind
  CL^2 : Math  Operator=square  SaturateOnIntegerOverflow=on
  Constant terms : Constant  Value=as.CD0
  Sum : Sum  Inputs=|+-  SaturateOnIntegerOverflow=on  InputSameDT=on  OutDataTypeStr=Inherit: Same as first input
  Sum1 : Sum  Inputs=++++  SaturateOnIntegerOverflow=on  InputSameDT=on  OutDataTypeStr=Inherit: Same as first input
  CD : Outport
  wires:
  Constant terms/1 -> Sum1/1
  CDdf/1 -> Sum1/2
  CDM/1 -> Sum1/3
  Abs4/1 -> CDdf/1
  control/1 -> Abs4/1
  Mach/1 -> CDM/1
  Sum1/1 -> CD/1  "CD"
  CL^2/1 -> (CL-CL0)^2/(pi e AR)/1
  Sum/1 -> CL^2/1
  CL/1 -> Sum/1
  CL min drag/1 -> Sum/2
  (CL-CL0)^2/(pi e AR)/1 -> Sum1/4

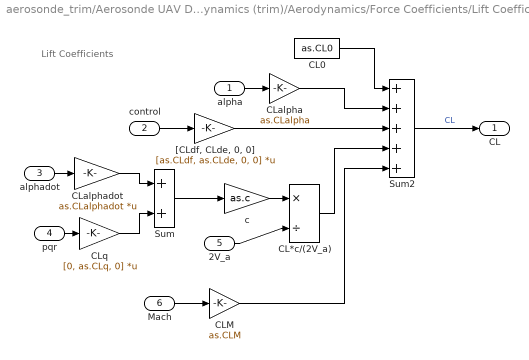
== system aerosonde_trim/Aerosonde UAV Dynamics (trim)/Aerodynamics/Force Coefficients/Lift Coefficients ==
  note: Lift Coefficients
  alpha : Inport
  control : Inport  Port=2
  alphadot : Inport  Port=3
  pqr : Inport  Port=4
  2V_a : Inport  Port=5
  Mach : Inport  Port=6
  CL*c/(2V_a) : Product  Inputs=*/  SaturateOnIntegerOverflow=on  InputSameDT=on  OutDataTypeStr=Inherit: Same as first input
  CL0 : Constant  Value=as.CL0
  CLM : Gain  Gain=as.CLM  SaturateOnIntegerOverflow=on  OutDataTypeStr=Inherit: Same as input  ParamDataTypeStr=Inherit: Same as input
  CLalpha : Gain  Gain=as.CLalpha  SaturateOnIntegerOverflow=on  OutDataTypeStr=Inherit: Same as input  ParamDataTypeStr=Inherit: Same as input
  CLalphadot : Gain  Gain=as.CLalphadot  Multiplication=Matrix(K*u)  SaturateOnIntegerOverflow=on  OutDataTypeStr=Inherit: Same as input  ParamDataTypeStr=Inherit: Same as input
  CLq : Gain  Gain=[0, as.CLq, 0]  Multiplication=Matrix(K*u)  SaturateOnIntegerOverflow=on  OutDataTypeStr=Inherit: Same as input  ParamDataTypeStr=Inherit: Same as input
  Sum : Sum  SaturateOnIntegerOverflow=on  InputSameDT=on  OutDataTypeStr=Inherit: Same as first input
  Sum2 : Sum  Inputs=+++++  SaturateOnIntegerOverflow=on  InputSameDT=on  OutDataTypeStr=Inherit: Same as first input
  "[CLdf, CLde, 0, 0]" : Gain  Gain=[as.CLdf, as.CLde, 0, 0]  Multiplication=Matrix(K*u)  SaturateOnIntegerOverflow=on  OutDataTypeStr=Inherit: Same as input  ParamDataTypeStr=Inherit: Same as input
  c : Gain  Gain=as.c  SaturateOnIntegerOverflow=on  OutDataTypeStr=Inherit: Same as input  ParamDataTypeStr=Inherit: Same as input
  CL : Outport
  wires:
  CLq/1 -> Sum/2
  CLalphadot/1 -> Sum/1
  Sum/1 -> c/1
  CL0/1 -> Sum2/1
  CLalpha/1 -> Sum2/2
  "[CLdf, CLde, 0, 0]"/1 -> Sum2/3
  Sum2/1 -> CL/1  "CL"
  CLM/1 -> Sum2/5
  CL*c/(2V_a)/1 -> Sum2/4
  c/1 -> CL*c/(2V_a)/1
  control/1 -> "[CLdf, CLde, 0, 0]"/1
  pqr/1 -> CLq/1
  2V_a/1 -> CL*c/(2V_a)/2
  Mach/1 -> CLM/1
  alpha/1 -> CLalpha/1
  alphadot/1 -> CLalphadot/1

== system aerosonde_trim/Aerosonde UAV Dynamics (trim)/Aerodynamics/Force Coefficients/Side Force Coefficients ==
  note: Side force coefficients
  beta : Inport
  control : Inport  Port=2
  angular rates : Inport  Port=3
  2V_a : Inport  Port=4
  CY*b/(2V_a) : Product  Inputs=*/  SaturateOnIntegerOverflow=on  InputSameDT=on  OutDataTypeStr=Inherit: Same as first input
  CYbeta : Gain  Gain=as.CYbeta  SaturateOnIntegerOverflow=on  OutDataTypeStr=Inherit: Same as input  ParamDataTypeStr=Inherit: Same as input
  Sum3 : Sum  Inputs=+++  SaturateOnIntegerOverflow=on  InputSameDT=on  OutDataTypeStr=Inherit: Same as first input
  Wing span1 : Gain  Gain=as.b  SaturateOnIntegerOverflow=on  OutDataTypeStr=Inherit: Same as input  ParamDataTypeStr=Inherit: Same as input
  "[0, 0, CYda, CYdr]" : Gain  Gain=[0, 0, as.CYda, as.CYdr]  Multiplication=Matrix(K*u)  SaturateOnIntegerOverflow=on  OutDataTypeStr=Inherit: Same as input  ParamDataTypeStr=Inherit: Same as input
  "[CYp, 0, CYr]" : Gain  Gain=[as.CYp, 0, as.CYr]  Multiplication=Matrix(K*u)  SaturateOnIntegerOverflow=on  OutDataTypeStr=Inherit: Same as input  ParamDataTypeStr=Inherit: Same as input
  CY : Outport
  wires:
  "[CYp, 0, CYr]"/1 -> Wing span1/1
  CYbeta/1 -> Sum3/1
  "[0, 0, CYda, CYdr]"/1 -> Sum3/2
  CY*b/(2V_a)/1 -> Sum3/3
  Sum3/1 -> CY/1  "CY"
  Wing span1/1 -> CY*b/(2V_a)/1
  control/1 -> "[0, 0, CYda, CYdr]"/1
  angular rates/1 -> "[CYp, 0, CYr]"/1
  2V_a/1 -> CY*b/(2V_a)/2
  beta/1 -> CYbeta/1

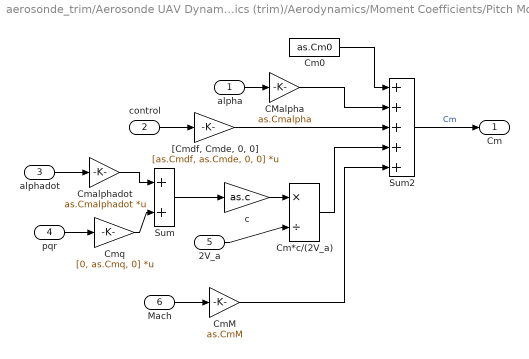
== system aerosonde_trim/Aerosonde UAV Dynamics (trim)/Aerodynamics/Moment Coefficients/Pitch Moment Coefficients ==
  alpha : Inport
  control : Inport  Port=2
  alphadot : Inport  Port=3
  pqr : Inport  Port=4
  2V_a : Inport  Port=5
  Mach : Inport  Port=6
  CMalpha : Gain  Gain=as.Cmalpha  SaturateOnIntegerOverflow=on  OutDataTypeStr=Inherit: Same as input  ParamDataTypeStr=Inherit: Same as input
  Cm*c/(2V_a) : Product  Inputs=*/  SaturateOnIntegerOverflow=on  InputSameDT=on  OutDataTypeStr=Inherit: Same as first input
  Cm0 : Constant  Value=as.Cm0
  CmM : Gain  Gain=as.CmM  SaturateOnIntegerOverflow=on  OutDataTypeStr=Inherit: Same as input  ParamDataTypeStr=Inherit: Same as input
  Cmalphadot : Gain  Gain=as.Cmalphadot  Multiplication=Matrix(K*u)  SaturateOnIntegerOverflow=on  OutDataTypeStr=Inherit: Same as input  ParamDataTypeStr=Inherit: Same as input
  Cmq : Gain  Gain=[0, as.Cmq, 0]  Multiplication=Matrix(K*u)  SaturateOnIntegerOverflow=on  OutDataTypeStr=Inherit: Same as input  ParamDataTypeStr=Inherit: Same as input
  Sum : Sum  SaturateOnIntegerOverflow=on  InputSameDT=on  OutDataTypeStr=Inherit: Same as first input
  Sum2 : Sum  Inputs=+++++  SaturateOnIntegerOverflow=on  InputSameDT=on  OutDataTypeStr=Inherit: Same as first input
  "[Cmdf, Cmde, 0, 0]" : Gain  Gain=[as.Cmdf, as.Cmde, 0, 0]  Multiplication=Matrix(K*u)  SaturateOnIntegerOverflow=on  OutDataTypeStr=Inherit: Same as input  ParamDataTypeStr=Inherit: Same as input
  c : Gain  Gain=as.c  SaturateOnIntegerOverflow=on  OutDataTypeStr=Inherit: Same as input  ParamDataTypeStr=Inherit: Same as input
  Cm : Outport
  wires:
  alphadot/1 -> Cmalphadot/1
  alpha/1 -> CMalpha/1
  Mach/1 -> CmM/1
  2V_a/1 -> Cm*c/(2V_a)/2
  pqr/1 -> Cmq/1
  control/1 -> "[Cmdf, Cmde, 0, 0]"/1
  c/1 -> Cm*c/(2V_a)/1
  Cm*c/(2V_a)/1 -> Sum2/4
  CmM/1 -> Sum2/5
  Sum2/1 -> Cm/1  "Cm"
  "[Cmdf, Cmde, 0, 0]"/1 -> Sum2/3
  CMalpha/1 -> Sum2/2
  Cm0/1 -> Sum2/1
  Sum/1 -> c/1
  Cmalphadot/1 -> Sum/1
  Cmq/1 -> Sum/2

== system aerosonde_trim/Aerosonde UAV Dynamics (trim)/Aerodynamics/Moment Coefficients/Roll Moment Coefficients ==
  note: Roll moment coefficient
  beta : Inport
  control : Inport  Port=2
  angular rates : Inport  Port=3
  2V : Inport  Port=4
  CY*b/(2V) : Product  Inputs=*/  SaturateOnIntegerOverflow=on  InputSameDT=on  OutDataTypeStr=Inherit: Same as first input
  Clbeta : Gain  Gain=as.Clbeta  SaturateOnIntegerOverflow=on  OutDataTypeStr=Inherit: Same as input  ParamDataTypeStr=Inherit: Same as input
  Sum3 : Sum  Inputs=+++  SaturateOnIntegerOverflow=on  InputSameDT=on  OutDataTypeStr=Inherit: Same as first input
  Wing span : Gain  Gain=as.b  SaturateOnIntegerOverflow=on  OutDataTypeStr=Inherit: Same as input  ParamDataTypeStr=Inherit: Same as input
  "[0, 0, Clda, Cldr]" : Gain  Gain=[0, 0, as.Clda, as.Cldr]  Multiplication=Matrix(K*u)  SaturateOnIntegerOverflow=on  OutDataTypeStr=Inherit: Same as input  ParamDataTypeStr=Inherit: Same as input
  "[Clp, 0, Clr]" : Gain  Gain=[as.Clp, 0, as.Clr]  Multiplication=Matrix(K*u)  SaturateOnIntegerOverflow=on  OutDataTypeStr=Inherit: Same as input  ParamDataTypeStr=Inherit: Same as input
  Cl : Outport
  wires:
  beta/1 -> Clbeta/1
  2V/1 -> CY*b/(2V)/2
  angular rates/1 -> "[Clp, 0, Clr]"/1
  control/1 -> "[0, 0, Clda, Cldr]"/1
  Wing span/1 -> CY*b/(2V)/1
  Sum3/1 -> Cl/1  "Cl"
  CY*b/(2V)/1 -> Sum3/3
  "[0, 0, Clda, Cldr]"/1 -> Sum3/2
  Clbeta/1 -> Sum3/1
  "[Clp, 0, Clr]"/1 -> Wing span/1

== system aerosonde_trim/Aerosonde UAV Dynamics (trim)/Aerodynamics/Moment Coefficients/Yaw Moment Coefficients ==
  note: Yaw moment coefficient
  beta : Inport
  control : Inport  Port=2
  angular rates : Inport  Port=3
  2V_a : Inport  Port=4
  Cn*b/(2V_a) : Product  Inputs=*/  SaturateOnIntegerOverflow=on  InputSameDT=on  OutDataTypeStr=Inherit: Same as first input
  Cnbeta : Gain  Gain=as.Cnbeta  SaturateOnIntegerOverflow=on  OutDataTypeStr=Inherit: Same as input  ParamDataTypeStr=Inherit: Same as input
  Sum3 : Sum  Inputs=+++  SaturateOnIntegerOverflow=on  InputSameDT=on  OutDataTypeStr=Inherit: Same as first input
  Wing span : Gain  Gain=as.b  SaturateOnIntegerOverflow=on  OutDataTypeStr=Inherit: Same as input  ParamDataTypeStr=Inherit: Same as input
  "[0, 0, Cnda, Cndr]" : Gain  Gain=[0, 0, as.Cnda, as.Cndr]  Multiplication=Matrix(K*u)  SaturateOnIntegerOverflow=on  OutDataTypeStr=Inherit: Same as input  ParamDataTypeStr=Inherit: Same as input
  "[Cnp, 0, Cnr]" : Gain  Gain=[as.Cnp, 0, as.Cnr]  Multiplication=Matrix(K*u)  SaturateOnIntegerOverflow=on  OutDataTypeStr=Inherit: Same as input  ParamDataTypeStr=Inherit: Same as input
  Cn : Outport
  wires:
  "[Cnp, 0, Cnr]"/1 -> Wing span/1
  Cnbeta/1 -> Sum3/1
  "[0, 0, Cnda, Cndr]"/1 -> Sum3/2
  Cn*b/(2V_a)/1 -> Sum3/3
  Sum3/1 -> Cn/1  "Cn"
  Wing span/1 -> Cn*b/(2V_a)/1
  control/1 -> "[0, 0, Cnda, Cndr]"/1
  angular rates/1 -> "[Cnp, 0, Cnr]"/1
  2V_a/1 -> Cn*b/(2V_a)/2
  beta/1 -> Cnbeta/1

== system aerosonde_trim/Aerosonde UAV Dynamics (trim)/Aerodynamics/Wind-axes Velocities (with algebraic loops broken)/Calculate  alphadot ==
  note: W
  note: Calculate alphadot
  "[Udot Vdot Wdot]" : Inport
  "[U V W]" : Inport  Port=2
  Demux : Demux  Outputs=3
  Demux1 : Demux  Outputs=3
  Math Function : Math  Operator=square  SaturateOnIntegerOverflow=on
  Math Function1 : Math  Operator=square  SaturateOnIntegerOverflow=on
  Product : Product  RndMeth=Zero
  Product1 : Product  RndMeth=Zero
  Product2 : Product  Inputs=*/  RndMeth=Zero
  Sum : Sum  Inputs=-|+
  Sum1 : Sum  Inputs=+|+
  Terminator : Terminator
  Terminator1 : Terminator
  alphadot : Outport
  wires:
  Demux/1 -> Product1/1  "Udot"
  Demux/3 -> Product/1  "Wdot"
  Demux/2 -> Terminator/1
  Demux1/1 -> Product/2, Math Function/1  "U"
  Demux1/3 -> Product1/2, Math Function1/1
  Math Function/1 -> Sum1/1
  Math Function1/1 -> Sum1/2
  Sum1/1 -> Product2/2  "U^2 + W^2"
  Product1/1 -> Sum/1  "W Udot"
  Product/1 -> Sum/2  "U Wdot"
  Sum/1 -> Product2/1
  Demux1/2 -> Terminator1/1
  "[U V W]"/1 -> Demux1/1
  "[Udot Vdot Wdot]"/1 -> Demux/1
  Product2/1 -> alphadot/1  "alphadot"

== system aerosonde_trim/Aerosonde UAV Dynamics (trim)/Propulsion System/Piston Engine/Altitude correction  for  Power ==
  note: Altitude correction for Power
  T : Inport
  Math Function : Math  Operator=sqrt  SaturateOnIntegerOverflow=on
  Product of Elements : Product  Inputs=/
  "Sea-level temperature " : Gain  Gain=TSL  SaturateOnIntegerOverflow=on  OutDataTypeStr=Inherit: Same as input  ParamDataTypeStr=Inherit: Same as input
  Power correction : Outport
  wires:
  Product of Elements/1 -> "Sea-level temperature "/1
  "Sea-level temperature "/1 -> Math Function/1
  Math Function/1 -> Power correction/1
  T/1 -> Product of Elements/1

== system aerosonde_trim/Aerosonde UAV Dynamics (trim)/Propulsion System/Piston Engine/Intake ==
  Thr : Inport  OutDataTypeStr=double  PortDimensions=1  DataType=double
  P_atm : Inport  Port=2  OutDataTypeStr=double  PortDimensions=1  DataType=double
  Get MAP : Product  SaturateOnIntegerOverflow=on  InputSameDT=on  OutDataTypeStr=Inherit: Same as first input
  MAP min : Constant  Value=as.MAPmin
  Saturation : Saturate  UpperLimit=inf  LowerLimit=as.MAPmin
  Sum : Sum  Inputs=|+-  SaturateOnIntegerOverflow=on  InputSameDT=on  OutDataTypeStr=Inherit: Same as first input
  Sum1 : Sum  Inputs=|++  SaturateOnIntegerOverflow=on  InputSameDT=on  OutDataTypeStr=Inherit: Same as first input
  kPa : Gain  Gain=1/1000  SaturateOnIntegerOverflow=on  OutDataTypeStr=Inherit: Same as input  ParamDataTypeStr=Inherit: Same as input
  MAP : Outport
  wires:
  Sum1/1 -> Saturation/1
  Get MAP/1 -> Sum1/1
  Sum/1 -> Get MAP/2
  kPa/1 -> Sum/1
  MAP min/1 -> Sum1/2, Sum/2
  Thr/1 -> Get MAP/1
  P_atm/1 -> kPa/1
  Saturation/1 -> MAP/1
